simulink model "Actuator_Control"  (R2015a)
settings: Solver=ode4  StartTime=0.0  StopTime=3  FixedStep=1e-6  RelTol=1e-3
libraries: simulink x1, aerolibactuator x1
settings Model: Creator=Jack  LastModifiedBy=Jack

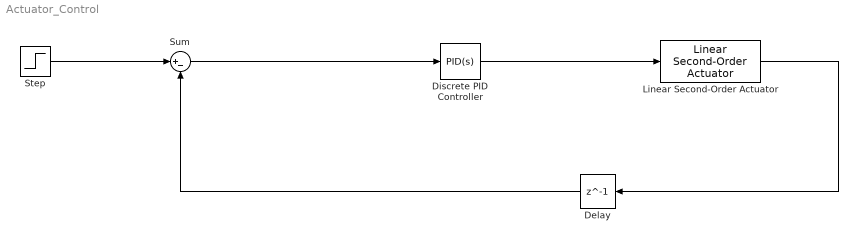
== system Actuator_Control ==
  Delay : Delay  DelayLength=1  InitialCondition=0
  Discrete PID Controller : simulink/Continuous/PID Controller  Controller=PID  TimeDomain=Continuous-time  SampleTime=-1  IntegratorMethod=Forward Euler  FilterMethod=Forward Euler  Form=Parallel  UseFilter=on  ControllerParametersSource=internal  P=4.51203991129563  I=17.5007609656002  D=0.220052873876515  N=3240.55689296992  InitialConditionSource=internal  InitialConditionForIntegrator=0  InitialConditionForFilter=0  ExternalReset=none  LimitOutput=on  UpperSaturationLimit=0.02  LowerSaturationLimit=-0.02  LinearizeAsGain=off  AntiWindupMode=none  Kb=1  TrackingMode=off  Kt=1  PParamMin=[]  PParamMax=[]  IParamMin=[]  IParamMax=[]  DParamMin=[]  DParamMax=[]  NParamMin=[]  NParamMax=[]  KbParamMin=[]  KbParamMax=[]  KtParamMin=[]  KtParamMax=[]  POutMin=[]  POutMax=[]  IOutMin=[]  IOutMax=[]  DOutMin=[]  DOutMax=[]  NOutMin=[]  NOutMax=[]  KbOutMin=[]  KbOutMax=[]  KtOutMin=[]  KtOutMax=[]  IntegratorOutMin=[]  IntegratorOutMax=[]  FilterOutMin=[]  FilterOutMax=[]  SumOutMin=[]  SumOutMax=[]  SumI1OutMin=[]  SumI1OutMax=[]  SumI2OutMin=[]  SumI2OutMax=[]  SumI3OutMin=[]  SumI3OutMax=[]  SumDOutMin=[]  SumDOutMax=[]  SaturationOutMin=[]  SaturationOutMax=[]  IntegratorContinuousStateAttributes=''  IntegratorStateMustResolveToSignalObject=off  IntegratorRTWStateStorageClass=Auto  FilterContinuousStateAttributes=''  FilterStateMustResolveToSignalObject=off  FilterRTWStateStorageClass=Auto  DifferentiatorICPrevScaledInput=0  DifferentiatorOutMin=[]  DifferentiatorOutMax=[]
  Linear Second-Order Actuator : aerolibactuator/Linear Second-Order Actuator  wn_fin=10  z_fin=0.3  fin_act_0=0  fin_act_vel=0
  Step : Step  After=0.01  SampleTime=0
  Sum : Sum  Inputs=|+-
  wires:
  Linear Second-Order Actuator/1 -> Delay/1
  Delay/1 -> Sum/2
  Sum/1 -> Discrete PID Controller/1
  Discrete PID Controller/1 -> Linear Second-Order Actuator/1
  Step/1 -> Sum/1
